simulink model "Controllers"  (R2023a)
settings: Solver=VariableStepAuto  StartTime=0.0  StopTime=10  RelTol=1e-3
values from neighbouring files (symbols this model uses):
  Gpz_den = Gpz.Denominator{1,1}    [deimian.m]
  Gpz_num = Gpz.Numerator{1,1}    [deimian.m]
  Kdz = (Kp*Taud)/T    (= 62.7240538515)    [deimian.m]
  Kiz = (Kp*T)/Taui    (= 42.7148147579)    [deimian.m]
  Kpz = Kp - (Kp * T)/(2*Taui)    (= 144.229508103)    [deimian.m]
  T = 0.05    [deimian.m]
undefined symbols (not defined in the file or in its folder): DiscIntNeverNeededParam, Gcz_db_den, Gcz_db_num, Gcz_den_dahlin, Gcz_num_dahlin
libraries: simulink x1
settings Model: Creator=maxpr  LastModifiedBy=maxpr

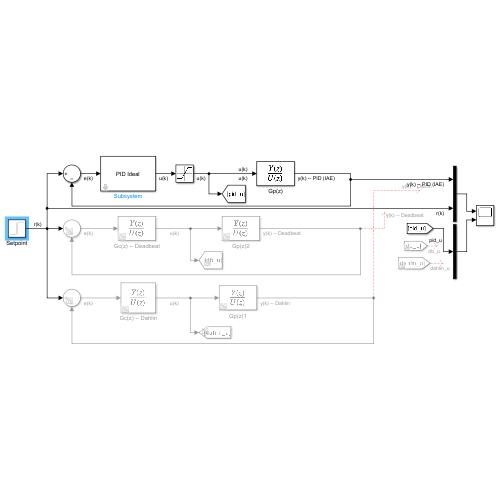
[thumbnail: Simulink's stored preview of the top-level diagram]
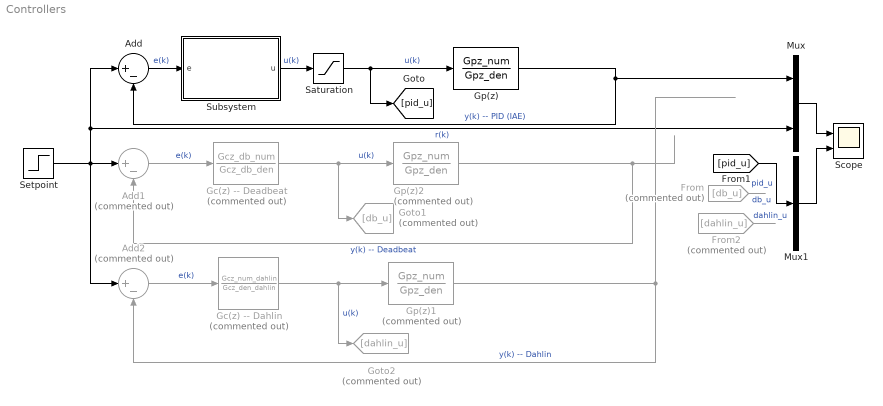
== system Controllers ==
  Add : Sum  Inputs=|+-
  Add1 : Sum  Commented=on  Inputs=|+-
  Add2 : Sum  Commented=on  Inputs=|+-
  From : From  Commented=on  GotoTag=db_u
  From2 : From  Commented=on  GotoTag=dahlin_u
  "Gc(z) -- Dahlin" : DiscreteTransferFcn  Commented=on  Numerator=Gcz_num_dahlin  Denominator=Gcz_den_dahlin  SampleTime=T
  "Gc(z) -- Deadbeat" : DiscreteTransferFcn  Commented=on  Numerator=Gcz_db_num  Denominator=Gcz_db_den  SampleTime=T
  Goto1 : Goto  Commented=on  GotoTag=db_u
  Goto2 : Goto  Commented=on  GotoTag=dahlin_u
  Gp(z) : DiscreteTransferFcn  Numerator=Gpz_num  Denominator=Gpz_den  SampleTime=T
  Gp(z)1 : DiscreteTransferFcn  Commented=on  Numerator=Gpz_num  Denominator=Gpz_den  SampleTime=T
  Gp(z)2 : DiscreteTransferFcn  Commented=on  Numerator=Gpz_num  Denominator=Gpz_den  SampleTime=T
  Mux : Mux  Inputs=2
  Mux1 : Mux  Inputs=1
  Saturation : Saturate  UpperLimit=255  LowerLimit=0
  Scope : Scope  NumInputPorts=2
  Setpoint : Step  Time=.05  After=2  SampleTime=T
  Subsystem : Subsystem  mask{Kp=Kpz, Ki=Kiz, Kd=Kdz}
      mask prompts: Kp "Ganancia proporcional"; Ki "Ganancia integral"; Kd "Ganancia derivativa"
      mask DialogControl ParameterGroupVar Prompt: PID params
      mask Display: disp('PID Ideal');
  wires:
  Add1/1 -> "Gc(z) -- Deadbeat"/1  "e(k)"
  Gp(z)2/1 -> Add1/2  "y(k) -- Deadbeat"
  Mux/1 -> Scope/1
  Mux1/1 -> Scope/2
  "Gc(z) -- Deadbeat"/1 -> Gp(z)2/1, Goto1/1  "u(k)"
  [pid_u] -> Mux1/1  "pid_u"
  From/1 -> ?  "db_u"
  Setpoint/1 -> Add2/1, Add/1, Mux/2, Add1/1  "r(k)"
  Gp(z)1/1 -> Add2/2  "y(k) -- Dahlin"
  Add2/1 -> "Gc(z) -- Dahlin"/1  "e(k)"
  "Gc(z) -- Dahlin"/1 -> Gp(z)1/1, Goto2/1  "u(k)"
  From2/1 -> ?  "dahlin_u"
  Gp(z)/1 -> Add/2, Mux/1  "y(k) -- PID (IAE)"
  Add/1 -> Subsystem/1(e)  "e(k)"
  Saturation/1 -> Gp(z)/1, [pid_u]  "u(k)"
  Subsystem/1(u) -> Saturation/1  "u(k)"

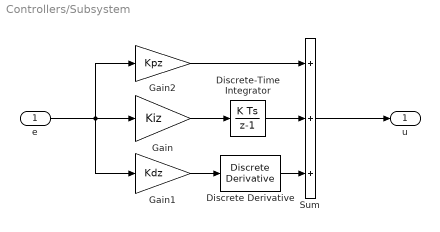
== system Controllers/Subsystem ==
  e : Inport
  Discrete Derivative : simulink/Discrete/Discrete Derivative  gainval=1.0  ICPrevScaledInput=0.0  OutMin=[]  OutMax=[]  OutDataType=fixdt(1, 16)  OutScaling=2^-10  DoSatur=off
  Discrete-Time Integrator : DiscreteIntegrator  SampleTime=T  ICPrevOutput=DiscIntNeverNeededParam  ICPrevScaledInput=DiscIntNeverNeededParam
  Gain : Gain  Gain=Kiz
  Gain1 : Gain  Gain=Kdz
  Gain2 : Gain  Gain=Kpz
  Sum : Sum  Inputs=+++
  u : Outport
  wires:
  e/1 -> Gain1/1, Gain/1, Gain2/1
  Sum/1 -> u/1
  Gain/1 -> Discrete-Time Integrator/1
  Gain1/1 -> Discrete Derivative/1
  Discrete Derivative/1 -> Sum/3
  Gain2/1 -> Sum/1
  Discrete-Time Integrator/1 -> Sum/2
